simulink model "Control_Loop4_2Model"  (R2013b)
settings: Solver=ode45  StartTime=0.0  StopTime=200  RelTol=1e-3
libraries: commutil2 x756, xpclib x100, etargetslib x98, dspnetwork x98, powerlib_meascontrol x24, commcrc2 x14, dspadpt3 x4, simulink_extras x4, dspmtrx3 x4, simulink x1
(part 5 of 7)

== system Control_Loop4_2Model/GISOO-Simulation Environment/SkyMote11/Triggered Subsystem ==
  In2 : Inport
  Trigger : TriggerPort
  Byte Reversal1 : etargetslib/Byte Reversal  numInp=1
  Data Type Conversion1 : DataTypeConversion  OutDataTypeStr=uint32
  Pack : xpclib/UDP/Pack  datatypes={'uint32'}  byteAlign=1
  UDP Send : dspnetwork/UDP Send  remoteURL='127.0.0.1'  remotePort=18000+moteID  localURL='0.0.0.0'  localPortSource=Automatically determine  localPort=-1  sampletime=-1  separateLengthPort=0
  wires:
  Data Type Conversion1/1 -> Byte Reversal1/1
  Byte Reversal1/1 -> Pack/1
  Pack/1 -> UDP Send/1
  In2/1 -> Data Type Conversion1/1

== system Control_Loop4_2Model/GISOO-Simulation Environment/SkyMote11/Triggered Subsystem1 ==
  In2 : Inport
  Trigger : TriggerPort
  Byte Reversal1 : etargetslib/Byte Reversal  numInp=1
  Data Type Conversion1 : DataTypeConversion  OutDataTypeStr=uint32
  Pack : xpclib/UDP/Pack  datatypes={'uint32'}  byteAlign=1
  UDP Send : dspnetwork/UDP Send  remoteURL='127.0.0.1'  remotePort=18000+moteID  localURL='0.0.0.0'  localPortSource=Automatically determine  localPort=-1  sampletime=-1  separateLengthPort=0
  wires:
  Byte Reversal1/1 -> Pack/1
  Data Type Conversion1/1 -> Byte Reversal1/1
  In2/1 -> Data Type Conversion1/1
  Pack/1 -> UDP Send/1

== system Control_Loop4_2Model/GISOO-Simulation Environment/SkyMote11/Triggered Subsystem2 ==
  In2 : Inport
  Trigger : TriggerPort
  Byte Reversal : etargetslib/Byte Reversal  numInp=1
  Data Type Conversion1 : DataTypeConversion  OutDataTypeStr=uint32
  Pack : xpclib/UDP/Pack  datatypes={'uint32'}  byteAlign=1
  UDP Send : dspnetwork/UDP Send  remoteURL='127.0.0.1'  remotePort=18000+moteID  localURL='0.0.0.0'  localPortSource=Automatically determine  localPort=-1  sampletime=-1  separateLengthPort=0
  Out1 : Outport
  wires:
  Byte Reversal/1 -> Pack/1
  Pack/1 -> UDP Send/1
  Data Type Conversion1/1 -> Byte Reversal/1, Out1/1
  In2/1 -> Data Type Conversion1/1

== system Control_Loop4_2Model/GISOO-Simulation Environment/SkyMote11/Triggered Subsystem3 ==
  In2 : Inport
  Trigger : TriggerPort
  Byte Reversal : etargetslib/Byte Reversal  numInp=1
  Data Type Conversion1 : DataTypeConversion  OutDataTypeStr=uint32
  Pack : xpclib/UDP/Pack  datatypes={'uint32'}  byteAlign=1
  UDP Send : dspnetwork/UDP Send  remoteURL='127.0.0.1'  remotePort=18000+moteID  localURL='0.0.0.0'  localPortSource=Automatically determine  localPort=-1  sampletime=-1  separateLengthPort=0
  Out1 : Outport
  wires:
  Byte Reversal/1 -> Pack/1
  In2/1 -> Data Type Conversion1/1
  Data Type Conversion1/1 -> Out1/1, Byte Reversal/1
  Pack/1 -> UDP Send/1

== system Control_Loop4_2Model/GISOO-Simulation Environment/SkyMote11/Triggered Subsystem4 ==
  RecivedSD : Inport
  Trigger : TriggerPort
  Byte Reversal : etargetslib/Byte Reversal  numInp=1
  Constant : Constant  Value=1111
  Data Type Conversion1 : DataTypeConversion  OutDataTypeStr=uint32
  Pack : xpclib/UDP/Pack  datatypes={'uint32'}  byteAlign=1
  UDP Send : dspnetwork/UDP Send  remoteURL='127.0.0.1'  remotePort=18000+moteID  localURL='0.0.0.0'  localPortSource=Automatically determine  localPort=-1  sampletime=-1  separateLengthPort=0
  SDToApplay : Outport
  wires:
  Data Type Conversion1/1 -> Byte Reversal/1
  Byte Reversal/1 -> Pack/1
  Constant/1 -> Data Type Conversion1/1
  RecivedSD/1 -> SDToApplay/1
  Pack/1 -> UDP Send/1

== system Control_Loop4_2Model/GISOO-Simulation Environment/SkyMote11/Triggered Subsystem5 ==
  SerialDataToSend : Inport
  Trigger : TriggerPort
  Byte Reversal : etargetslib/Byte Reversal  numInp=1
  Demux : Demux  Outputs=30
  Pack : xpclib/UDP/Pack  datatypes={'uint8','uint8','uint8','uint8','uint8','uint8','uint8','uint8','uint8','uint8','uint8','uint8','uint8','uint8','uint8','uint8','uint8','uint8','uint8','uint8','uint8','uint8','uint8','uint8','uint8','uint8','uint8','uint8','uint8','uint8'}  byteAlign=1
  UDP Send : dspnetwork/UDP Send  remoteURL='127.0.0.1'  remotePort=18000+moteID  localURL='0.0.0.0'  localPortSource=Automatically determine  localPort=-1  sampletime=-1  separateLengthPort=0
  wires:
  Pack/1 -> UDP Send/1
  Demux/1 -> Pack/1
  Demux/2 -> Pack/2
  Demux/3 -> Pack/3
  Demux/4 -> Pack/4
  Demux/5 -> Pack/5
  Demux/6 -> Pack/6
  Demux/7 -> Pack/7
  Demux/8 -> Pack/8
  Demux/9 -> Pack/9
  Demux/10 -> Pack/10
  Demux/11 -> Pack/11
  Demux/12 -> Pack/12
  Demux/13 -> Pack/13
  Demux/14 -> Pack/14
  Demux/15 -> Pack/15
  Demux/16 -> Pack/16
  Demux/17 -> Pack/17
  Demux/18 -> Pack/18
  Demux/19 -> Pack/19
  Demux/20 -> Pack/20
  Demux/21 -> Pack/21
  Demux/22 -> Pack/22
  Demux/23 -> Pack/23
  Demux/24 -> Pack/24
  Demux/25 -> Pack/25
  Demux/26 -> Pack/26
  Demux/27 -> Pack/27
  Demux/28 -> Pack/28
  Demux/29 -> Pack/29
  Demux/30 -> Pack/30
  SerialDataToSend/1 -> Byte Reversal/1
  Byte Reversal/1 -> Demux/1

== system Control_Loop4_2Model/GISOO-Simulation Environment/SkyMote12/ADC0 Sender ==
  In2 : Inport
  Trigger : TriggerPort
  Byte Reversal1 : etargetslib/Byte Reversal  numInp=1
  Data Type Conversion1 : DataTypeConversion  OutDataTypeStr=uint32
  Pack : xpclib/UDP/Pack  datatypes={'uint32'}  byteAlign=1
  UDP Send : dspnetwork/UDP Send  remoteURL='127.0.0.1'  remotePort=18000+moteID  localURL='0.0.0.0'  localPortSource=Automatically determine  localPort=-1  sampletime=-1  separateLengthPort=0
  wires:
  Data Type Conversion1/1 -> Byte Reversal1/1
  Byte Reversal1/1 -> Pack/1
  In2/1 -> Data Type Conversion1/1
  Pack/1 -> UDP Send/1

== system Control_Loop4_2Model/GISOO-Simulation Environment/SkyMote12/Subsystem ==
  SerialData : Inport
  AM Packet type : Constant  Value=PacketType  OutDataTypeStr=double
  Bit to Integer Converter{,1..27} (28 alike) : commutil2/Bit to Integer Converter  nbits=8  bitOrder=MSB first  signedOutputValues=Unsigned  outDtype=Inherit via internal rule  outDtypeSigned=Inherit via internal rule
  Constant25 : Constant  Value=72  OutDataTypeStr=double
  Constant26 : Constant  Value=0  OutDataTypeStr=double
  Constant{27..30} (4 alike) : Constant  Value=255  OutDataTypeStr=double
  Constant31 : Constant  Value=16  OutDataTypeStr=double
  Constant32 : Constant  Value=137  OutDataTypeStr=double
  Demux1 : Demux  Outputs=28
  Demux2 : Demux  Outputs=16
  FrameByteEnd : Constant  Value=126  OutDataTypeStr=uint8
  FrameByteStart : Constant  Value=126  OutDataTypeStr=uint8
  Framing byte : Constant  Value=68  OutDataTypeStr=uint8
  General CRC Generator1 : commcrc2/General CRC Generator  genPoly=[1 0 0 0 1 0 0 0 0 0 0 1 0 0 0 0 1]  iniStates=0  directMethod=off  reflectInputBytes=off  reflectChecksums=off  finalXOR=0  numChecksums=1
  Integer to Bit Converter{,1..25} (26 alike) : commutil2/Integer to Bit Converter  nbits=8  signedInputValues=Unsigned  bitOrder=MSB first  outDtype=boolean
  Mux1 : Mux  Inputs=26
  Mux2 : Mux  Inputs=30
  SerialFrame : Outport
  wires:
  Bit to Integer Converter27/1 -> Mux2/3
  Demux1/28 -> Bit to Integer Converter27/1
  FrameByteStart/1 -> Mux2/30
  Bit to Integer Converter26/1 -> Mux2/2
  Demux1/27 -> Bit to Integer Converter26/1
  Demux1/15 -> Bit to Integer Converter18/1
  Demux1/14 -> Bit to Integer Converter13/1
  Demux1/6 -> Bit to Integer Converter5/1
  Demux1/16 -> Bit to Integer Converter19/1
  Demux1/25 -> Bit to Integer Converter22/1
  Demux1/17 -> Bit to Integer Converter14/1
  Demux1/18 -> Bit to Integer Converter15/1
  Demux1/26 -> Bit to Integer Converter23/1
  Demux1/22 -> Bit to Integer Converter25/1
  Demux1/23 -> Bit to Integer Converter20/1
  Demux1/20 -> Bit to Integer Converter17/1
  Demux1/19 -> Bit to Integer Converter16/1
  Demux1/5 -> Bit to Integer Converter4/1
  Demux1/21 -> Bit to Integer Converter24/1
  Demux1/4 -> Bit to Integer Converter3/1
  Demux1/24 -> Bit to Integer Converter21/1
  Constant31/1 -> Integer to Bit Converter7/1
  Integer to Bit Converter19/1 -> Mux1/20
  Integer to Bit Converter20/1 -> Mux1/21
  Integer to Bit Converter9/1 -> Mux1/10
  Integer to Bit Converter18/1 -> Mux1/19
  Demux1/12 -> Bit to Integer Converter11/1
  Mux2/1 -> SerialFrame/1
  Integer to Bit Converter12/1 -> Mux1/13
  Demux2/9 -> Integer to Bit Converter18/1
  Demux1/7 -> Bit to Integer Converter6/1
  Demux1/13 -> Bit to Integer Converter12/1
  Demux1/9 -> Bit to Integer Converter8/1
  Demux1/1 -> Bit to Integer Converter/1
  Demux2/11 -> Integer to Bit Converter20/1
  Demux1/11 -> Bit to Integer Converter10/1
  AM Packet type/1 -> Integer to Bit Converter9/1
  FrameByteEnd/1 -> Mux2/1
  Integer to Bit Converter22/1 -> Mux1/23
  Integer to Bit Converter21/1 -> Mux1/22
  Integer to Bit Converter25/1 -> Mux1/26
  Constant32/1 -> Integer to Bit Converter8/1
  Integer to Bit Converter8/1 -> Mux1/9
  General CRC Generator1/1 -> Demux1/1
  Integer to Bit Converter7/1 -> Mux1/8
  Demux1/3 -> Bit to Integer Converter2/1
  Integer to Bit Converter2/1 -> Mux1/3
  Integer to Bit Converter3/1 -> Mux1/4
  Constant28/1 -> Integer to Bit Converter4/1
  Integer to Bit Converter4/1 -> Mux1/5
  Constant27/1 -> Integer to Bit Converter3/1
  Constant26/1 -> Integer to Bit Converter2/1
  Constant29/1 -> Integer to Bit Converter5/1
  Integer to Bit Converter1/1 -> Mux1/2
  Integer to Bit Converter5/1 -> Mux1/6
  Demux2/14 -> Integer to Bit Converter23/1
  Demux2/16 -> Integer to Bit Converter25/1
  Mux1/1 -> General CRC Generator1/1
  Framing byte/1 -> Integer to Bit Converter/1
  Demux2/15 -> Integer to Bit Converter24/1
  Demux2/13 -> Integer to Bit Converter22/1
  Integer to Bit Converter/1 -> Mux1/1
  Demux2/12 -> Integer to Bit Converter21/1
  Constant25/1 -> Integer to Bit Converter1/1
  Demux2/8 -> Integer to Bit Converter17/1
  Integer to Bit Converter10/1 -> Mux1/11
  Demux2/10 -> Integer to Bit Converter19/1
  Integer to Bit Converter6/1 -> Mux1/7
  Demux1/2 -> Bit to Integer Converter1/1
  Integer to Bit Converter16/1 -> Mux1/17
  Integer to Bit Converter15/1 -> Mux1/16
  Integer to Bit Converter17/1 -> Mux1/18
  Integer to Bit Converter13/1 -> Mux1/14
  Demux1/8 -> Bit to Integer Converter7/1
  Demux1/10 -> Bit to Integer Converter9/1
  Constant30/1 -> Integer to Bit Converter6/1
  Integer to Bit Converter11/1 -> Mux1/12
  Integer to Bit Converter23/1 -> Mux1/24
  Integer to Bit Converter24/1 -> Mux1/25
  Integer to Bit Converter14/1 -> Mux1/15
  Demux2/6 -> Integer to Bit Converter15/1
  Demux2/5 -> Integer to Bit Converter14/1
  Bit to Integer Converter22/1 -> Mux2/5
  SerialData/1 -> Demux2/1
  Bit to Integer Converter21/1 -> Mux2/6
  Demux2/2 -> Integer to Bit Converter11/1
  Demux2/1 -> Integer to Bit Converter10/1
  Bit to Integer Converter17/1 -> Mux2/10
  Bit to Integer Converter20/1 -> Mux2/7
  Bit to Integer Converter/1 -> Mux2/29
  Bit to Integer Converter9/1 -> Mux2/20
  Bit to Integer Converter7/1 -> Mux2/22
  Bit to Integer Converter11/1 -> Mux2/18
  Bit to Integer Converter4/1 -> Mux2/25
  Bit to Integer Converter1/1 -> Mux2/28
  Bit to Integer Converter6/1 -> Mux2/23
  Bit to Integer Converter10/1 -> Mux2/19
  Bit to Integer Converter25/1 -> Mux2/8
  Bit to Integer Converter15/1 -> Mux2/12
  Bit to Integer Converter13/1 -> Mux2/16
  Bit to Integer Converter16/1 -> Mux2/11
  Bit to Integer Converter2/1 -> Mux2/27
  Bit to Integer Converter5/1 -> Mux2/24
  Demux2/7 -> Integer to Bit Converter16/1
  Bit to Integer Converter14/1 -> Mux2/13
  Bit to Integer Converter19/1 -> Mux2/14
  Bit to Integer Converter12/1 -> Mux2/17
  Bit to Integer Converter18/1 -> Mux2/15
  Demux2/3 -> Integer to Bit Converter12/1
  Bit to Integer Converter8/1 -> Mux2/21
  Bit to Integer Converter24/1 -> Mux2/9
  Demux2/4 -> Integer to Bit Converter13/1
  Bit to Integer Converter3/1 -> Mux2/26
  Bit to Integer Converter23/1 -> Mux2/4

== system Control_Loop4_2Model/GISOO-Simulation Environment/SkyMote12/Triggered Subsystem ==
  In2 : Inport
  Trigger : TriggerPort
  Byte Reversal1 : etargetslib/Byte Reversal  numInp=1
  Data Type Conversion1 : DataTypeConversion  OutDataTypeStr=uint32
  Pack : xpclib/UDP/Pack  datatypes={'uint32'}  byteAlign=1
  UDP Send : dspnetwork/UDP Send  remoteURL='127.0.0.1'  remotePort=18000+moteID  localURL='0.0.0.0'  localPortSource=Automatically determine  localPort=-1  sampletime=-1  separateLengthPort=0
  wires:
  Data Type Conversion1/1 -> Byte Reversal1/1
  Byte Reversal1/1 -> Pack/1
  Pack/1 -> UDP Send/1
  In2/1 -> Data Type Conversion1/1

== system Control_Loop4_2Model/GISOO-Simulation Environment/SkyMote12/Triggered Subsystem1 ==
  In2 : Inport
  Trigger : TriggerPort
  Byte Reversal1 : etargetslib/Byte Reversal  numInp=1
  Data Type Conversion1 : DataTypeConversion  OutDataTypeStr=uint32
  Pack : xpclib/UDP/Pack  datatypes={'uint32'}  byteAlign=1
  UDP Send : dspnetwork/UDP Send  remoteURL='127.0.0.1'  remotePort=18000+moteID  localURL='0.0.0.0'  localPortSource=Automatically determine  localPort=-1  sampletime=-1  separateLengthPort=0
  wires:
  Byte Reversal1/1 -> Pack/1
  Data Type Conversion1/1 -> Byte Reversal1/1
  In2/1 -> Data Type Conversion1/1
  Pack/1 -> UDP Send/1

== system Control_Loop4_2Model/GISOO-Simulation Environment/SkyMote12/Triggered Subsystem2 ==
  In2 : Inport
  Trigger : TriggerPort
  Byte Reversal : etargetslib/Byte Reversal  numInp=1
  Data Type Conversion1 : DataTypeConversion  OutDataTypeStr=uint32
  Pack : xpclib/UDP/Pack  datatypes={'uint32'}  byteAlign=1
  UDP Send : dspnetwork/UDP Send  remoteURL='127.0.0.1'  remotePort=18000+moteID  localURL='0.0.0.0'  localPortSource=Automatically determine  localPort=-1  sampletime=-1  separateLengthPort=0
  Out1 : Outport
  wires:
  Byte Reversal/1 -> Pack/1
  Pack/1 -> UDP Send/1
  Data Type Conversion1/1 -> Byte Reversal/1, Out1/1
  In2/1 -> Data Type Conversion1/1

== system Control_Loop4_2Model/GISOO-Simulation Environment/SkyMote12/Triggered Subsystem3 ==
  In2 : Inport
  Trigger : TriggerPort
  Byte Reversal : etargetslib/Byte Reversal  numInp=1
  Data Type Conversion1 : DataTypeConversion  OutDataTypeStr=uint32
  Pack : xpclib/UDP/Pack  datatypes={'uint32'}  byteAlign=1
  UDP Send : dspnetwork/UDP Send  remoteURL='127.0.0.1'  remotePort=18000+moteID  localURL='0.0.0.0'  localPortSource=Automatically determine  localPort=-1  sampletime=-1  separateLengthPort=0
  Out1 : Outport
  wires:
  Byte Reversal/1 -> Pack/1
  In2/1 -> Data Type Conversion1/1
  Data Type Conversion1/1 -> Out1/1, Byte Reversal/1
  Pack/1 -> UDP Send/1

== system Control_Loop4_2Model/GISOO-Simulation Environment/SkyMote12/Triggered Subsystem4 ==
  RecivedSD : Inport
  Trigger : TriggerPort
  Byte Reversal : etargetslib/Byte Reversal  numInp=1
  Constant : Constant  Value=1111
  Data Type Conversion1 : DataTypeConversion  OutDataTypeStr=uint32
  Pack : xpclib/UDP/Pack  datatypes={'uint32'}  byteAlign=1
  UDP Send : dspnetwork/UDP Send  remoteURL='127.0.0.1'  remotePort=18000+moteID  localURL='0.0.0.0'  localPortSource=Automatically determine  localPort=-1  sampletime=-1  separateLengthPort=0
  SDToApplay : Outport
  wires:
  Data Type Conversion1/1 -> Byte Reversal/1
  Byte Reversal/1 -> Pack/1
  Constant/1 -> Data Type Conversion1/1
  RecivedSD/1 -> SDToApplay/1
  Pack/1 -> UDP Send/1

== system Control_Loop4_2Model/GISOO-Simulation Environment/SkyMote12/Triggered Subsystem5 ==
  SerialDataToSend : Inport
  Trigger : TriggerPort
  Byte Reversal : etargetslib/Byte Reversal  numInp=1
  Demux : Demux  Outputs=30
  Pack : xpclib/UDP/Pack  datatypes={'uint8','uint8','uint8','uint8','uint8','uint8','uint8','uint8','uint8','uint8','uint8','uint8','uint8','uint8','uint8','uint8','uint8','uint8','uint8','uint8','uint8','uint8','uint8','uint8','uint8','uint8','uint8','uint8','uint8','uint8'}  byteAlign=1
  UDP Send : dspnetwork/UDP Send  remoteURL='127.0.0.1'  remotePort=18000+moteID  localURL='0.0.0.0'  localPortSource=Automatically determine  localPort=-1  sampletime=-1  separateLengthPort=0
  wires:
  Pack/1 -> UDP Send/1
  Demux/1 -> Pack/1
  Demux/2 -> Pack/2
  Demux/3 -> Pack/3
  Demux/4 -> Pack/4
  Demux/5 -> Pack/5
  Demux/6 -> Pack/6
  Demux/7 -> Pack/7
  Demux/8 -> Pack/8
  Demux/9 -> Pack/9
  Demux/10 -> Pack/10
  Demux/11 -> Pack/11
  Demux/12 -> Pack/12
  Demux/13 -> Pack/13
  Demux/14 -> Pack/14
  Demux/15 -> Pack/15
  Demux/16 -> Pack/16
  Demux/17 -> Pack/17
  Demux/18 -> Pack/18
  Demux/19 -> Pack/19
  Demux/20 -> Pack/20
  Demux/21 -> Pack/21
  Demux/22 -> Pack/22
  Demux/23 -> Pack/23
  Demux/24 -> Pack/24
  Demux/25 -> Pack/25
  Demux/26 -> Pack/26
  Demux/27 -> Pack/27
  Demux/28 -> Pack/28
  Demux/29 -> Pack/29
  Demux/30 -> Pack/30
  SerialDataToSend/1 -> Byte Reversal/1
  Byte Reversal/1 -> Demux/1

== system Control_Loop4_2Model/GISOO-Simulation Environment/SkyMote13/ADC0 Sender ==
  In2 : Inport
  Trigger : TriggerPort
  Byte Reversal1 : etargetslib/Byte Reversal  numInp=1
  Data Type Conversion1 : DataTypeConversion  OutDataTypeStr=uint32
  Pack : xpclib/UDP/Pack  datatypes={'uint32'}  byteAlign=1
  UDP Send : dspnetwork/UDP Send  remoteURL='127.0.0.1'  remotePort=18000+moteID  localURL='0.0.0.0'  localPortSource=Automatically determine  localPort=-1  sampletime=-1  separateLengthPort=0
  wires:
  Data Type Conversion1/1 -> Byte Reversal1/1
  Byte Reversal1/1 -> Pack/1
  In2/1 -> Data Type Conversion1/1
  Pack/1 -> UDP Send/1

== system Control_Loop4_2Model/GISOO-Simulation Environment/SkyMote13/Subsystem ==
  SerialData : Inport
  AM Packet type : Constant  Value=PacketType  OutDataTypeStr=double
  Bit to Integer Converter{,1..27} (28 alike) : commutil2/Bit to Integer Converter  nbits=8  bitOrder=MSB first  signedOutputValues=Unsigned  outDtype=Inherit via internal rule  outDtypeSigned=Inherit via internal rule
  Constant25 : Constant  Value=72  OutDataTypeStr=double
  Constant26 : Constant  Value=0  OutDataTypeStr=double
  Constant{27..30} (4 alike) : Constant  Value=255  OutDataTypeStr=double
  Constant31 : Constant  Value=16  OutDataTypeStr=double
  Constant32 : Constant  Value=137  OutDataTypeStr=double
  Demux1 : Demux  Outputs=28
  Demux2 : Demux  Outputs=16
  FrameByteEnd : Constant  Value=126  OutDataTypeStr=uint8
  FrameByteStart : Constant  Value=126  OutDataTypeStr=uint8
  Framing byte : Constant  Value=68  OutDataTypeStr=uint8
  General CRC Generator1 : commcrc2/General CRC Generator  genPoly=[1 0 0 0 1 0 0 0 0 0 0 1 0 0 0 0 1]  iniStates=0  directMethod=off  reflectInputBytes=off  reflectChecksums=off  finalXOR=0  numChecksums=1
  Integer to Bit Converter{,1..25} (26 alike) : commutil2/Integer to Bit Converter  nbits=8  signedInputValues=Unsigned  bitOrder=MSB first  outDtype=boolean
  Mux1 : Mux  Inputs=26
  Mux2 : Mux  Inputs=30
  SerialFrame : Outport
  wires:
  Bit to Integer Converter27/1 -> Mux2/3
  Demux1/28 -> Bit to Integer Converter27/1
  FrameByteStart/1 -> Mux2/30
  Bit to Integer Converter26/1 -> Mux2/2
  Demux1/27 -> Bit to Integer Converter26/1
  Demux1/15 -> Bit to Integer Converter18/1
  Demux1/14 -> Bit to Integer Converter13/1
  Demux1/6 -> Bit to Integer Converter5/1
  Demux1/16 -> Bit to Integer Converter19/1
  Demux1/25 -> Bit to Integer Converter22/1
  Demux1/17 -> Bit to Integer Converter14/1
  Demux1/18 -> Bit to Integer Converter15/1
  Demux1/26 -> Bit to Integer Converter23/1
  Demux1/22 -> Bit to Integer Converter25/1
  Demux1/23 -> Bit to Integer Converter20/1
  Demux1/20 -> Bit to Integer Converter17/1
  Demux1/19 -> Bit to Integer Converter16/1
  Demux1/5 -> Bit to Integer Converter4/1
  Demux1/21 -> Bit to Integer Converter24/1
  Demux1/4 -> Bit to Integer Converter3/1
  Demux1/24 -> Bit to Integer Converter21/1
  Constant31/1 -> Integer to Bit Converter7/1
  Integer to Bit Converter19/1 -> Mux1/20
  Integer to Bit Converter20/1 -> Mux1/21
  Integer to Bit Converter9/1 -> Mux1/10
  Integer to Bit Converter18/1 -> Mux1/19
  Demux1/12 -> Bit to Integer Converter11/1
  Mux2/1 -> SerialFrame/1
  Integer to Bit Converter12/1 -> Mux1/13
  Demux2/9 -> Integer to Bit Converter18/1
  Demux1/7 -> Bit to Integer Converter6/1
  Demux1/13 -> Bit to Integer Converter12/1
  Demux1/9 -> Bit to Integer Converter8/1
  Demux1/1 -> Bit to Integer Converter/1
  Demux2/11 -> Integer to Bit Converter20/1
  Demux1/11 -> Bit to Integer Converter10/1
  AM Packet type/1 -> Integer to Bit Converter9/1
  FrameByteEnd/1 -> Mux2/1
  Integer to Bit Converter22/1 -> Mux1/23
  Integer to Bit Converter21/1 -> Mux1/22
  Integer to Bit Converter25/1 -> Mux1/26
  Constant32/1 -> Integer to Bit Converter8/1
  Integer to Bit Converter8/1 -> Mux1/9
  General CRC Generator1/1 -> Demux1/1
  Integer to Bit Converter7/1 -> Mux1/8
  Demux1/3 -> Bit to Integer Converter2/1
  Integer to Bit Converter2/1 -> Mux1/3
  Integer to Bit Converter3/1 -> Mux1/4
  Constant28/1 -> Integer to Bit Converter4/1
  Integer to Bit Converter4/1 -> Mux1/5
  Constant27/1 -> Integer to Bit Converter3/1
  Constant26/1 -> Integer to Bit Converter2/1
  Constant29/1 -> Integer to Bit Converter5/1
  Integer to Bit Converter1/1 -> Mux1/2
  Integer to Bit Converter5/1 -> Mux1/6
  Demux2/14 -> Integer to Bit Converter23/1
  Demux2/16 -> Integer to Bit Converter25/1
  Mux1/1 -> General CRC Generator1/1
  Framing byte/1 -> Integer to Bit Converter/1
  Demux2/15 -> Integer to Bit Converter24/1
  Demux2/13 -> Integer to Bit Converter22/1
  Integer to Bit Converter/1 -> Mux1/1
  Demux2/12 -> Integer to Bit Converter21/1
  Constant25/1 -> Integer to Bit Converter1/1
  Demux2/8 -> Integer to Bit Converter17/1
  Integer to Bit Converter10/1 -> Mux1/11
  Demux2/10 -> Integer to Bit Converter19/1
  Integer to Bit Converter6/1 -> Mux1/7
  Demux1/2 -> Bit to Integer Converter1/1
  Integer to Bit Converter16/1 -> Mux1/17
  Integer to Bit Converter15/1 -> Mux1/16
  Integer to Bit Converter17/1 -> Mux1/18
  Integer to Bit Converter13/1 -> Mux1/14
  Demux1/8 -> Bit to Integer Converter7/1
  Demux1/10 -> Bit to Integer Converter9/1
  Constant30/1 -> Integer to Bit Converter6/1
  Integer to Bit Converter11/1 -> Mux1/12
  Integer to Bit Converter23/1 -> Mux1/24
  Integer to Bit Converter24/1 -> Mux1/25
  Integer to Bit Converter14/1 -> Mux1/15
  Demux2/6 -> Integer to Bit Converter15/1
  Demux2/5 -> Integer to Bit Converter14/1
  Bit to Integer Converter22/1 -> Mux2/5
  SerialData/1 -> Demux2/1
  Bit to Integer Converter21/1 -> Mux2/6
  Demux2/2 -> Integer to Bit Converter11/1
  Demux2/1 -> Integer to Bit Converter10/1
  Bit to Integer Converter17/1 -> Mux2/10
  Bit to Integer Converter20/1 -> Mux2/7
  Bit to Integer Converter/1 -> Mux2/29
  Bit to Integer Converter9/1 -> Mux2/20
  Bit to Integer Converter7/1 -> Mux2/22
  Bit to Integer Converter11/1 -> Mux2/18
  Bit to Integer Converter4/1 -> Mux2/25
  Bit to Integer Converter1/1 -> Mux2/28
  Bit to Integer Converter6/1 -> Mux2/23
  Bit to Integer Converter10/1 -> Mux2/19
  Bit to Integer Converter25/1 -> Mux2/8
  Bit to Integer Converter15/1 -> Mux2/12
  Bit to Integer Converter13/1 -> Mux2/16
  Bit to Integer Converter16/1 -> Mux2/11
  Bit to Integer Converter2/1 -> Mux2/27
  Bit to Integer Converter5/1 -> Mux2/24
  Demux2/7 -> Integer to Bit Converter16/1
  Bit to Integer Converter14/1 -> Mux2/13
  Bit to Integer Converter19/1 -> Mux2/14
  Bit to Integer Converter12/1 -> Mux2/17
  Bit to Integer Converter18/1 -> Mux2/15
  Demux2/3 -> Integer to Bit Converter12/1
  Bit to Integer Converter8/1 -> Mux2/21
  Bit to Integer Converter24/1 -> Mux2/9
  Demux2/4 -> Integer to Bit Converter13/1
  Bit to Integer Converter3/1 -> Mux2/26
  Bit to Integer Converter23/1 -> Mux2/4

== system Control_Loop4_2Model/GISOO-Simulation Environment/SkyMote13/Triggered Subsystem ==
  In2 : Inport
  Trigger : TriggerPort
  Byte Reversal1 : etargetslib/Byte Reversal  numInp=1
  Data Type Conversion1 : DataTypeConversion  OutDataTypeStr=uint32
  Pack : xpclib/UDP/Pack  datatypes={'uint32'}  byteAlign=1
  UDP Send : dspnetwork/UDP Send  remoteURL='127.0.0.1'  remotePort=18000+moteID  localURL='0.0.0.0'  localPortSource=Automatically determine  localPort=-1  sampletime=-1  separateLengthPort=0
  wires:
  Data Type Conversion1/1 -> Byte Reversal1/1
  Byte Reversal1/1 -> Pack/1
  Pack/1 -> UDP Send/1
  In2/1 -> Data Type Conversion1/1

== system Control_Loop4_2Model/GISOO-Simulation Environment/SkyMote13/Triggered Subsystem1 ==
  In2 : Inport
  Trigger : TriggerPort
  Byte Reversal1 : etargetslib/Byte Reversal  numInp=1
  Data Type Conversion1 : DataTypeConversion  OutDataTypeStr=uint32
  Pack : xpclib/UDP/Pack  datatypes={'uint32'}  byteAlign=1
  UDP Send : dspnetwork/UDP Send  remoteURL='127.0.0.1'  remotePort=18000+moteID  localURL='0.0.0.0'  localPortSource=Automatically determine  localPort=-1  sampletime=-1  separateLengthPort=0
  wires:
  Byte Reversal1/1 -> Pack/1
  Data Type Conversion1/1 -> Byte Reversal1/1
  In2/1 -> Data Type Conversion1/1
  Pack/1 -> UDP Send/1

== system Control_Loop4_2Model/GISOO-Simulation Environment/SkyMote13/Triggered Subsystem2 ==
  In2 : Inport
  Trigger : TriggerPort
  Byte Reversal : etargetslib/Byte Reversal  numInp=1
  Data Type Conversion1 : DataTypeConversion  OutDataTypeStr=uint32
  Pack : xpclib/UDP/Pack  datatypes={'uint32'}  byteAlign=1
  UDP Send : dspnetwork/UDP Send  remoteURL='127.0.0.1'  remotePort=18000+moteID  localURL='0.0.0.0'  localPortSource=Automatically determine  localPort=-1  sampletime=-1  separateLengthPort=0
  Out1 : Outport
  wires:
  Byte Reversal/1 -> Pack/1
  Pack/1 -> UDP Send/1
  Data Type Conversion1/1 -> Byte Reversal/1, Out1/1
  In2/1 -> Data Type Conversion1/1

== system Control_Loop4_2Model/GISOO-Simulation Environment/SkyMote13/Triggered Subsystem3 ==
  In2 : Inport
  Trigger : TriggerPort
  Byte Reversal : etargetslib/Byte Reversal  numInp=1
  Data Type Conversion1 : DataTypeConversion  OutDataTypeStr=uint32
  Pack : xpclib/UDP/Pack  datatypes={'uint32'}  byteAlign=1
  UDP Send : dspnetwork/UDP Send  remoteURL='127.0.0.1'  remotePort=18000+moteID  localURL='0.0.0.0'  localPortSource=Automatically determine  localPort=-1  sampletime=-1  separateLengthPort=0
  Out1 : Outport
  wires:
  Byte Reversal/1 -> Pack/1
  In2/1 -> Data Type Conversion1/1
  Data Type Conversion1/1 -> Out1/1, Byte Reversal/1
  Pack/1 -> UDP Send/1

== system Control_Loop4_2Model/GISOO-Simulation Environment/SkyMote13/Triggered Subsystem4 ==
  RecivedSD : Inport
  Trigger : TriggerPort
  Byte Reversal : etargetslib/Byte Reversal  numInp=1
  Constant : Constant  Value=1111
  Data Type Conversion1 : DataTypeConversion  OutDataTypeStr=uint32
  Pack : xpclib/UDP/Pack  datatypes={'uint32'}  byteAlign=1
  UDP Send : dspnetwork/UDP Send  remoteURL='127.0.0.1'  remotePort=18000+moteID  localURL='0.0.0.0'  localPortSource=Automatically determine  localPort=-1  sampletime=-1  separateLengthPort=0
  SDToApplay : Outport
  wires:
  Data Type Conversion1/1 -> Byte Reversal/1
  Byte Reversal/1 -> Pack/1
  Constant/1 -> Data Type Conversion1/1
  RecivedSD/1 -> SDToApplay/1
  Pack/1 -> UDP Send/1

== system Control_Loop4_2Model/GISOO-Simulation Environment/SkyMote13/Triggered Subsystem5 ==
  SerialDataToSend : Inport
  Trigger : TriggerPort
  Byte Reversal : etargetslib/Byte Reversal  numInp=1
  Demux : Demux  Outputs=30
  Pack : xpclib/UDP/Pack  datatypes={'uint8','uint8','uint8','uint8','uint8','uint8','uint8','uint8','uint8','uint8','uint8','uint8','uint8','uint8','uint8','uint8','uint8','uint8','uint8','uint8','uint8','uint8','uint8','uint8','uint8','uint8','uint8','uint8','uint8','uint8'}  byteAlign=1
  UDP Send : dspnetwork/UDP Send  remoteURL='127.0.0.1'  remotePort=18000+moteID  localURL='0.0.0.0'  localPortSource=Automatically determine  localPort=-1  sampletime=-1  separateLengthPort=0
  wires:
  Pack/1 -> UDP Send/1
  Demux/1 -> Pack/1
  Demux/2 -> Pack/2
  Demux/3 -> Pack/3
  Demux/4 -> Pack/4
  Demux/5 -> Pack/5
  Demux/6 -> Pack/6
  Demux/7 -> Pack/7
  Demux/8 -> Pack/8
  Demux/9 -> Pack/9
  Demux/10 -> Pack/10
  Demux/11 -> Pack/11
  Demux/12 -> Pack/12
  Demux/13 -> Pack/13
  Demux/14 -> Pack/14
  Demux/15 -> Pack/15
  Demux/16 -> Pack/16
  Demux/17 -> Pack/17
  Demux/18 -> Pack/18
  Demux/19 -> Pack/19
  Demux/20 -> Pack/20
  Demux/21 -> Pack/21
  Demux/22 -> Pack/22
  Demux/23 -> Pack/23
  Demux/24 -> Pack/24
  Demux/25 -> Pack/25
  Demux/26 -> Pack/26
  Demux/27 -> Pack/27
  Demux/28 -> Pack/28
  Demux/29 -> Pack/29
  Demux/30 -> Pack/30
  SerialDataToSend/1 -> Byte Reversal/1
  Byte Reversal/1 -> Demux/1

== system Control_Loop4_2Model/GISOO-Simulation Environment/SkyMote2/ADC0 Sender ==
  In2 : Inport
  Trigger : TriggerPort
  Byte Reversal1 : etargetslib/Byte Reversal  numInp=1
  Data Type Conversion1 : DataTypeConversion  OutDataTypeStr=uint32
  Pack : xpclib/UDP/Pack  datatypes={'uint32'}  byteAlign=1
  UDP Send : dspnetwork/UDP Send  remoteURL='127.0.0.1'  remotePort=18000+moteID  localURL='0.0.0.0'  localPortSource=Automatically determine  localPort=-1  sampletime=-1  separateLengthPort=0
  wires:
  Data Type Conversion1/1 -> Byte Reversal1/1
  Byte Reversal1/1 -> Pack/1
  In2/1 -> Data Type Conversion1/1
  Pack/1 -> UDP Send/1

== system Control_Loop4_2Model/GISOO-Simulation Environment/SkyMote2/Subsystem ==
  SerialData : Inport
  AM Packet type : Constant  Value=PacketType  OutDataTypeStr=double
  Bit to Integer Converter{,1..27} (28 alike) : commutil2/Bit to Integer Converter  nbits=8  bitOrder=MSB first  signedOutputValues=Unsigned  outDtype=Inherit via internal rule  outDtypeSigned=Inherit via internal rule
  Constant25 : Constant  Value=72  OutDataTypeStr=double
  Constant26 : Constant  Value=0  OutDataTypeStr=double
  Constant{27..30} (4 alike) : Constant  Value=255  OutDataTypeStr=double
  Constant31 : Constant  Value=16  OutDataTypeStr=double
  Constant32 : Constant  Value=137  OutDataTypeStr=double
  Demux1 : Demux  Outputs=28
  Demux2 : Demux  Outputs=16
  FrameByteEnd : Constant  Value=126  OutDataTypeStr=uint8
  FrameByteStart : Constant  Value=126  OutDataTypeStr=uint8
  Framing byte : Constant  Value=68  OutDataTypeStr=uint8
  General CRC Generator1 : commcrc2/General CRC Generator  genPoly=[1 0 0 0 1 0 0 0 0 0 0 1 0 0 0 0 1]  iniStates=0  directMethod=off  reflectInputBytes=off  reflectChecksums=off  finalXOR=0  numChecksums=1
  Integer to Bit Converter{,1..25} (26 alike) : commutil2/Integer to Bit Converter  nbits=8  signedInputValues=Unsigned  bitOrder=MSB first  outDtype=boolean
  Mux1 : Mux  Inputs=26
  Mux2 : Mux  Inputs=30
  SerialFrame : Outport
  wires:
  Bit to Integer Converter27/1 -> Mux2/3
  Demux1/28 -> Bit to Integer Converter27/1
  FrameByteStart/1 -> Mux2/30
  Bit to Integer Converter26/1 -> Mux2/2
  Demux1/27 -> Bit to Integer Converter26/1
  Demux1/15 -> Bit to Integer Converter18/1
  Demux1/14 -> Bit to Integer Converter13/1
  Demux1/6 -> Bit to Integer Converter5/1
  Demux1/16 -> Bit to Integer Converter19/1
  Demux1/25 -> Bit to Integer Converter22/1
  Demux1/17 -> Bit to Integer Converter14/1
  Demux1/18 -> Bit to Integer Converter15/1
  Demux1/26 -> Bit to Integer Converter23/1
  Demux1/22 -> Bit to Integer Converter25/1
  Demux1/23 -> Bit to Integer Converter20/1
  Demux1/20 -> Bit to Integer Converter17/1
  Demux1/19 -> Bit to Integer Converter16/1
  Demux1/5 -> Bit to Integer Converter4/1
  Demux1/21 -> Bit to Integer Converter24/1
  Demux1/4 -> Bit to Integer Converter3/1
  Demux1/24 -> Bit to Integer Converter21/1
  Constant31/1 -> Integer to Bit Converter7/1
  Integer to Bit Converter19/1 -> Mux1/20
  Integer to Bit Converter20/1 -> Mux1/21
  Integer to Bit Converter9/1 -> Mux1/10
  Integer to Bit Converter18/1 -> Mux1/19
  Demux1/12 -> Bit to Integer Converter11/1
  Mux2/1 -> SerialFrame/1
  Integer to Bit Converter12/1 -> Mux1/13
  Demux2/9 -> Integer to Bit Converter18/1
  Demux1/7 -> Bit to Integer Converter6/1
  Demux1/13 -> Bit to Integer Converter12/1
  Demux1/9 -> Bit to Integer Converter8/1
  Demux1/1 -> Bit to Integer Converter/1
  Demux2/11 -> Integer to Bit Converter20/1
  Demux1/11 -> Bit to Integer Converter10/1
  AM Packet type/1 -> Integer to Bit Converter9/1
  FrameByteEnd/1 -> Mux2/1
  Integer to Bit Converter22/1 -> Mux1/23
  Integer to Bit Converter21/1 -> Mux1/22
  Integer to Bit Converter25/1 -> Mux1/26
  Constant32/1 -> Integer to Bit Converter8/1
  Integer to Bit Converter8/1 -> Mux1/9
  General CRC Generator1/1 -> Demux1/1
  Integer to Bit Converter7/1 -> Mux1/8
  Demux1/3 -> Bit to Integer Converter2/1
  Integer to Bit Converter2/1 -> Mux1/3
  Integer to Bit Converter3/1 -> Mux1/4
  Constant28/1 -> Integer to Bit Converter4/1
  Integer to Bit Converter4/1 -> Mux1/5
  Constant27/1 -> Integer to Bit Converter3/1
  Constant26/1 -> Integer to Bit Converter2/1
  Constant29/1 -> Integer to Bit Converter5/1
  Integer to Bit Converter1/1 -> Mux1/2
  Integer to Bit Converter5/1 -> Mux1/6
  Demux2/14 -> Integer to Bit Converter23/1
  Demux2/16 -> Integer to Bit Converter25/1
  Mux1/1 -> General CRC Generator1/1
  Framing byte/1 -> Integer to Bit Converter/1
  Demux2/15 -> Integer to Bit Converter24/1
  Demux2/13 -> Integer to Bit Converter22/1
  Integer to Bit Converter/1 -> Mux1/1
  Demux2/12 -> Integer to Bit Converter21/1
  Constant25/1 -> Integer to Bit Converter1/1
  Demux2/8 -> Integer to Bit Converter17/1
  Integer to Bit Converter10/1 -> Mux1/11
  Demux2/10 -> Integer to Bit Converter19/1
  Integer to Bit Converter6/1 -> Mux1/7
  Demux1/2 -> Bit to Integer Converter1/1
  Integer to Bit Converter16/1 -> Mux1/17
  Integer to Bit Converter15/1 -> Mux1/16
  Integer to Bit Converter17/1 -> Mux1/18
  Integer to Bit Converter13/1 -> Mux1/14
  Demux1/8 -> Bit to Integer Converter7/1
  Demux1/10 -> Bit to Integer Converter9/1
  Constant30/1 -> Integer to Bit Converter6/1
  Integer to Bit Converter11/1 -> Mux1/12
  Integer to Bit Converter23/1 -> Mux1/24
  Integer to Bit Converter24/1 -> Mux1/25
  Integer to Bit Converter14/1 -> Mux1/15
  Demux2/6 -> Integer to Bit Converter15/1
  Demux2/5 -> Integer to Bit Converter14/1
  Bit to Integer Converter22/1 -> Mux2/5
  SerialData/1 -> Demux2/1
  Bit to Integer Converter21/1 -> Mux2/6
  Demux2/2 -> Integer to Bit Converter11/1
  Demux2/1 -> Integer to Bit Converter10/1
  Bit to Integer Converter17/1 -> Mux2/10
  Bit to Integer Converter20/1 -> Mux2/7
  Bit to Integer Converter/1 -> Mux2/29
  Bit to Integer Converter9/1 -> Mux2/20
  Bit to Integer Converter7/1 -> Mux2/22
  Bit to Integer Converter11/1 -> Mux2/18
  Bit to Integer Converter4/1 -> Mux2/25
  Bit to Integer Converter1/1 -> Mux2/28
  Bit to Integer Converter6/1 -> Mux2/23
  Bit to Integer Converter10/1 -> Mux2/19
  Bit to Integer Converter25/1 -> Mux2/8
  Bit to Integer Converter15/1 -> Mux2/12
  Bit to Integer Converter13/1 -> Mux2/16
  Bit to Integer Converter16/1 -> Mux2/11
  Bit to Integer Converter2/1 -> Mux2/27
  Bit to Integer Converter5/1 -> Mux2/24
  Demux2/7 -> Integer to Bit Converter16/1
  Bit to Integer Converter14/1 -> Mux2/13
  Bit to Integer Converter19/1 -> Mux2/14
  Bit to Integer Converter12/1 -> Mux2/17
  Bit to Integer Converter18/1 -> Mux2/15
  Demux2/3 -> Integer to Bit Converter12/1
  Bit to Integer Converter8/1 -> Mux2/21
  Bit to Integer Converter24/1 -> Mux2/9
  Demux2/4 -> Integer to Bit Converter13/1
  Bit to Integer Converter3/1 -> Mux2/26
  Bit to Integer Converter23/1 -> Mux2/4

== system Control_Loop4_2Model/GISOO-Simulation Environment/SkyMote2/Triggered Subsystem ==
  In2 : Inport
  Trigger : TriggerPort
  Byte Reversal1 : etargetslib/Byte Reversal  numInp=1
  Data Type Conversion1 : DataTypeConversion  OutDataTypeStr=uint32
  Pack : xpclib/UDP/Pack  datatypes={'uint32'}  byteAlign=1
  UDP Send : dspnetwork/UDP Send  remoteURL='127.0.0.1'  remotePort=18000+moteID  localURL='0.0.0.0'  localPortSource=Automatically determine  localPort=-1  sampletime=-1  separateLengthPort=0
  wires:
  Data Type Conversion1/1 -> Byte Reversal1/1
  Byte Reversal1/1 -> Pack/1
  Pack/1 -> UDP Send/1
  In2/1 -> Data Type Conversion1/1

== system Control_Loop4_2Model/GISOO-Simulation Environment/SkyMote2/Triggered Subsystem1 ==
  In2 : Inport
  Trigger : TriggerPort
  Byte Reversal1 : etargetslib/Byte Reversal  numInp=1
  Data Type Conversion1 : DataTypeConversion  OutDataTypeStr=uint32
  Pack : xpclib/UDP/Pack  datatypes={'uint32'}  byteAlign=1
  UDP Send : dspnetwork/UDP Send  remoteURL='127.0.0.1'  remotePort=18000+moteID  localURL='0.0.0.0'  localPortSource=Automatically determine  localPort=-1  sampletime=-1  separateLengthPort=0
  wires:
  Byte Reversal1/1 -> Pack/1
  Data Type Conversion1/1 -> Byte Reversal1/1
  In2/1 -> Data Type Conversion1/1
  Pack/1 -> UDP Send/1

== system Control_Loop4_2Model/GISOO-Simulation Environment/SkyMote2/Triggered Subsystem2 ==
  In2 : Inport
  Trigger : TriggerPort
  Byte Reversal : etargetslib/Byte Reversal  numInp=1
  Data Type Conversion1 : DataTypeConversion  OutDataTypeStr=uint32
  Pack : xpclib/UDP/Pack  datatypes={'uint32'}  byteAlign=1
  UDP Send : dspnetwork/UDP Send  remoteURL='127.0.0.1'  remotePort=18000+moteID  localURL='0.0.0.0'  localPortSource=Automatically determine  localPort=-1  sampletime=-1  separateLengthPort=0
  Out1 : Outport
  wires:
  Byte Reversal/1 -> Pack/1
  Pack/1 -> UDP Send/1
  Data Type Conversion1/1 -> Byte Reversal/1, Out1/1
  In2/1 -> Data Type Conversion1/1

== system Control_Loop4_2Model/GISOO-Simulation Environment/SkyMote2/Triggered Subsystem3 ==
  In2 : Inport
  Trigger : TriggerPort
  Byte Reversal : etargetslib/Byte Reversal  numInp=1
  Data Type Conversion1 : DataTypeConversion  OutDataTypeStr=uint32
  Pack : xpclib/UDP/Pack  datatypes={'uint32'}  byteAlign=1
  UDP Send : dspnetwork/UDP Send  remoteURL='127.0.0.1'  remotePort=18000+moteID  localURL='0.0.0.0'  localPortSource=Automatically determine  localPort=-1  sampletime=-1  separateLengthPort=0
  Out1 : Outport
  wires:
  Byte Reversal/1 -> Pack/1
  In2/1 -> Data Type Conversion1/1
  Data Type Conversion1/1 -> Out1/1, Byte Reversal/1
  Pack/1 -> UDP Send/1

== system Control_Loop4_2Model/GISOO-Simulation Environment/SkyMote2/Triggered Subsystem4 ==
  RecivedSD : Inport
  Trigger : TriggerPort
  Byte Reversal : etargetslib/Byte Reversal  numInp=1
  Constant : Constant  Value=1111
  Data Type Conversion1 : DataTypeConversion  OutDataTypeStr=uint32
  Pack : xpclib/UDP/Pack  datatypes={'uint32'}  byteAlign=1
  UDP Send : dspnetwork/UDP Send  remoteURL='127.0.0.1'  remotePort=18000+moteID  localURL='0.0.0.0'  localPortSource=Automatically determine  localPort=-1  sampletime=-1  separateLengthPort=0
  SDToApplay : Outport
  wires:
  Data Type Conversion1/1 -> Byte Reversal/1
  Byte Reversal/1 -> Pack/1
  Constant/1 -> Data Type Conversion1/1
  RecivedSD/1 -> SDToApplay/1
  Pack/1 -> UDP Send/1

== system Control_Loop4_2Model/GISOO-Simulation Environment/SkyMote2/Triggered Subsystem5 ==
  SerialDataToSend : Inport
  Trigger : TriggerPort
  Byte Reversal : etargetslib/Byte Reversal  numInp=1
  Demux : Demux  Outputs=30
  Pack : xpclib/UDP/Pack  datatypes={'uint8','uint8','uint8','uint8','uint8','uint8','uint8','uint8','uint8','uint8','uint8','uint8','uint8','uint8','uint8','uint8','uint8','uint8','uint8','uint8','uint8','uint8','uint8','uint8','uint8','uint8','uint8','uint8','uint8','uint8'}  byteAlign=1
  UDP Send : dspnetwork/UDP Send  remoteURL='127.0.0.1'  remotePort=18000+moteID  localURL='0.0.0.0'  localPortSource=Automatically determine  localPort=-1  sampletime=-1  separateLengthPort=0
  wires:
  Pack/1 -> UDP Send/1
  Demux/1 -> Pack/1
  Demux/2 -> Pack/2
  Demux/3 -> Pack/3
  Demux/4 -> Pack/4
  Demux/5 -> Pack/5
  Demux/6 -> Pack/6
  Demux/7 -> Pack/7
  Demux/8 -> Pack/8
  Demux/9 -> Pack/9
  Demux/10 -> Pack/10
  Demux/11 -> Pack/11
  Demux/12 -> Pack/12
  Demux/13 -> Pack/13
  Demux/14 -> Pack/14
  Demux/15 -> Pack/15
  Demux/16 -> Pack/16
  Demux/17 -> Pack/17
  Demux/18 -> Pack/18
  Demux/19 -> Pack/19
  Demux/20 -> Pack/20
  Demux/21 -> Pack/21
  Demux/22 -> Pack/22
  Demux/23 -> Pack/23
  Demux/24 -> Pack/24
  Demux/25 -> Pack/25
  Demux/26 -> Pack/26
  Demux/27 -> Pack/27
  Demux/28 -> Pack/28
  Demux/29 -> Pack/29
  Demux/30 -> Pack/30
  SerialDataToSend/1 -> Byte Reversal/1
  Byte Reversal/1 -> Demux/1

== system Control_Loop4_2Model/GISOO-Simulation Environment/SkyMote3/ADC0 Sender ==
  In2 : Inport
  Trigger : TriggerPort
  Byte Reversal1 : etargetslib/Byte Reversal  numInp=1
  Data Type Conversion1 : DataTypeConversion  OutDataTypeStr=uint32
  Pack : xpclib/UDP/Pack  datatypes={'uint32'}  byteAlign=1
  UDP Send : dspnetwork/UDP Send  remoteURL='127.0.0.1'  remotePort=18000+moteID  localURL='0.0.0.0'  localPortSource=Automatically determine  localPort=-1  sampletime=-1  separateLengthPort=0
  wires:
  Data Type Conversion1/1 -> Byte Reversal1/1
  Byte Reversal1/1 -> Pack/1
  In2/1 -> Data Type Conversion1/1
  Pack/1 -> UDP Send/1

== system Control_Loop4_2Model/GISOO-Simulation Environment/SkyMote3/Subsystem ==
  SerialData : Inport
  AM Packet type : Constant  Value=PacketType  OutDataTypeStr=double
  Bit to Integer Converter{,1..27} (28 alike) : commutil2/Bit to Integer Converter  nbits=8  bitOrder=MSB first  signedOutputValues=Unsigned  outDtype=Inherit via internal rule  outDtypeSigned=Inherit via internal rule
  Constant25 : Constant  Value=72  OutDataTypeStr=double
  Constant26 : Constant  Value=0  OutDataTypeStr=double
  Constant{27..30} (4 alike) : Constant  Value=255  OutDataTypeStr=double
  Constant31 : Constant  Value=16  OutDataTypeStr=double
  Constant32 : Constant  Value=137  OutDataTypeStr=double
  Demux1 : Demux  Outputs=28
  Demux2 : Demux  Outputs=16
  FrameByteEnd : Constant  Value=126  OutDataTypeStr=uint8
  FrameByteStart : Constant  Value=126  OutDataTypeStr=uint8
  Framing byte : Constant  Value=68  OutDataTypeStr=uint8
  General CRC Generator1 : commcrc2/General CRC Generator  genPoly=[1 0 0 0 1 0 0 0 0 0 0 1 0 0 0 0 1]  iniStates=0  directMethod=off  reflectInputBytes=off  reflectChecksums=off  finalXOR=0  numChecksums=1
  Integer to Bit Converter{,1..25} (26 alike) : commutil2/Integer to Bit Converter  nbits=8  signedInputValues=Unsigned  bitOrder=MSB first  outDtype=boolean
  Mux1 : Mux  Inputs=26
  Mux2 : Mux  Inputs=30
  SerialFrame : Outport
  wires:
  Bit to Integer Converter27/1 -> Mux2/3
  Demux1/28 -> Bit to Integer Converter27/1
  FrameByteStart/1 -> Mux2/30
  Bit to Integer Converter26/1 -> Mux2/2
  Demux1/27 -> Bit to Integer Converter26/1
  Demux1/15 -> Bit to Integer Converter18/1
  Demux1/14 -> Bit to Integer Converter13/1
  Demux1/6 -> Bit to Integer Converter5/1
  Demux1/16 -> Bit to Integer Converter19/1
  Demux1/25 -> Bit to Integer Converter22/1
  Demux1/17 -> Bit to Integer Converter14/1
  Demux1/18 -> Bit to Integer Converter15/1
  Demux1/26 -> Bit to Integer Converter23/1
  Demux1/22 -> Bit to Integer Converter25/1
  Demux1/23 -> Bit to Integer Converter20/1
  Demux1/20 -> Bit to Integer Converter17/1
  Demux1/19 -> Bit to Integer Converter16/1
  Demux1/5 -> Bit to Integer Converter4/1
  Demux1/21 -> Bit to Integer Converter24/1
  Demux1/4 -> Bit to Integer Converter3/1
  Demux1/24 -> Bit to Integer Converter21/1
  Constant31/1 -> Integer to Bit Converter7/1
  Integer to Bit Converter19/1 -> Mux1/20
  Integer to Bit Converter20/1 -> Mux1/21
  Integer to Bit Converter9/1 -> Mux1/10
  Integer to Bit Converter18/1 -> Mux1/19
  Demux1/12 -> Bit to Integer Converter11/1
  Mux2/1 -> SerialFrame/1
  Integer to Bit Converter12/1 -> Mux1/13
  Demux2/9 -> Integer to Bit Converter18/1
  Demux1/7 -> Bit to Integer Converter6/1
  Demux1/13 -> Bit to Integer Converter12/1
  Demux1/9 -> Bit to Integer Converter8/1
  Demux1/1 -> Bit to Integer Converter/1
  Demux2/11 -> Integer to Bit Converter20/1
  Demux1/11 -> Bit to Integer Converter10/1
  AM Packet type/1 -> Integer to Bit Converter9/1
  FrameByteEnd/1 -> Mux2/1
  Integer to Bit Converter22/1 -> Mux1/23
  Integer to Bit Converter21/1 -> Mux1/22
  Integer to Bit Converter25/1 -> Mux1/26
  Constant32/1 -> Integer to Bit Converter8/1
  Integer to Bit Converter8/1 -> Mux1/9
  General CRC Generator1/1 -> Demux1/1
  Integer to Bit Converter7/1 -> Mux1/8
  Demux1/3 -> Bit to Integer Converter2/1
  Integer to Bit Converter2/1 -> Mux1/3
  Integer to Bit Converter3/1 -> Mux1/4
  Constant28/1 -> Integer to Bit Converter4/1
  Integer to Bit Converter4/1 -> Mux1/5
  Constant27/1 -> Integer to Bit Converter3/1
  Constant26/1 -> Integer to Bit Converter2/1
  Constant29/1 -> Integer to Bit Converter5/1
  Integer to Bit Converter1/1 -> Mux1/2
  Integer to Bit Converter5/1 -> Mux1/6
  Demux2/14 -> Integer to Bit Converter23/1
  Demux2/16 -> Integer to Bit Converter25/1
  Mux1/1 -> General CRC Generator1/1
  Framing byte/1 -> Integer to Bit Converter/1
  Demux2/15 -> Integer to Bit Converter24/1
  Demux2/13 -> Integer to Bit Converter22/1
  Integer to Bit Converter/1 -> Mux1/1
  Demux2/12 -> Integer to Bit Converter21/1
  Constant25/1 -> Integer to Bit Converter1/1
  Demux2/8 -> Integer to Bit Converter17/1
  Integer to Bit Converter10/1 -> Mux1/11
  Demux2/10 -> Integer to Bit Converter19/1
  Integer to Bit Converter6/1 -> Mux1/7
  Demux1/2 -> Bit to Integer Converter1/1
  Integer to Bit Converter16/1 -> Mux1/17
  Integer to Bit Converter15/1 -> Mux1/16
  Integer to Bit Converter17/1 -> Mux1/18
  Integer to Bit Converter13/1 -> Mux1/14
  Demux1/8 -> Bit to Integer Converter7/1
  Demux1/10 -> Bit to Integer Converter9/1
  Constant30/1 -> Integer to Bit Converter6/1
  Integer to Bit Converter11/1 -> Mux1/12
  Integer to Bit Converter23/1 -> Mux1/24
  Integer to Bit Converter24/1 -> Mux1/25
  Integer to Bit Converter14/1 -> Mux1/15
  Demux2/6 -> Integer to Bit Converter15/1
  Demux2/5 -> Integer to Bit Converter14/1
  Bit to Integer Converter22/1 -> Mux2/5
  SerialData/1 -> Demux2/1
  Bit to Integer Converter21/1 -> Mux2/6
  Demux2/2 -> Integer to Bit Converter11/1
  Demux2/1 -> Integer to Bit Converter10/1
  Bit to Integer Converter17/1 -> Mux2/10
  Bit to Integer Converter20/1 -> Mux2/7
  Bit to Integer Converter/1 -> Mux2/29
  Bit to Integer Converter9/1 -> Mux2/20
  Bit to Integer Converter7/1 -> Mux2/22
  Bit to Integer Converter11/1 -> Mux2/18
  Bit to Integer Converter4/1 -> Mux2/25
  Bit to Integer Converter1/1 -> Mux2/28
  Bit to Integer Converter6/1 -> Mux2/23
  Bit to Integer Converter10/1 -> Mux2/19
  Bit to Integer Converter25/1 -> Mux2/8
  Bit to Integer Converter15/1 -> Mux2/12
  Bit to Integer Converter13/1 -> Mux2/16
  Bit to Integer Converter16/1 -> Mux2/11
  Bit to Integer Converter2/1 -> Mux2/27
  Bit to Integer Converter5/1 -> Mux2/24
  Demux2/7 -> Integer to Bit Converter16/1
  Bit to Integer Converter14/1 -> Mux2/13
  Bit to Integer Converter19/1 -> Mux2/14
  Bit to Integer Converter12/1 -> Mux2/17
  Bit to Integer Converter18/1 -> Mux2/15
  Demux2/3 -> Integer to Bit Converter12/1
  Bit to Integer Converter8/1 -> Mux2/21
  Bit to Integer Converter24/1 -> Mux2/9
  Demux2/4 -> Integer to Bit Converter13/1
  Bit to Integer Converter3/1 -> Mux2/26
  Bit to Integer Converter23/1 -> Mux2/4

== system Control_Loop4_2Model/GISOO-Simulation Environment/SkyMote3/Triggered Subsystem ==
  In2 : Inport
  Trigger : TriggerPort
  Byte Reversal1 : etargetslib/Byte Reversal  numInp=1
  Data Type Conversion1 : DataTypeConversion  OutDataTypeStr=uint32
  Pack : xpclib/UDP/Pack  datatypes={'uint32'}  byteAlign=1
  UDP Send : dspnetwork/UDP Send  remoteURL='127.0.0.1'  remotePort=18000+moteID  localURL='0.0.0.0'  localPortSource=Automatically determine  localPort=-1  sampletime=-1  separateLengthPort=0
  wires:
  Data Type Conversion1/1 -> Byte Reversal1/1
  Byte Reversal1/1 -> Pack/1
  Pack/1 -> UDP Send/1
  In2/1 -> Data Type Conversion1/1

== system Control_Loop4_2Model/GISOO-Simulation Environment/SkyMote3/Triggered Subsystem1 ==
  In2 : Inport
  Trigger : TriggerPort
  Byte Reversal1 : etargetslib/Byte Reversal  numInp=1
  Data Type Conversion1 : DataTypeConversion  OutDataTypeStr=uint32
  Pack : xpclib/UDP/Pack  datatypes={'uint32'}  byteAlign=1
  UDP Send : dspnetwork/UDP Send  remoteURL='127.0.0.1'  remotePort=18000+moteID  localURL='0.0.0.0'  localPortSource=Automatically determine  localPort=-1  sampletime=-1  separateLengthPort=0
  wires:
  Byte Reversal1/1 -> Pack/1
  Data Type Conversion1/1 -> Byte Reversal1/1
  In2/1 -> Data Type Conversion1/1
  Pack/1 -> UDP Send/1

== system Control_Loop4_2Model/GISOO-Simulation Environment/SkyMote3/Triggered Subsystem2 ==
  In2 : Inport
  Trigger : TriggerPort
  Byte Reversal : etargetslib/Byte Reversal  numInp=1
  Data Type Conversion1 : DataTypeConversion  OutDataTypeStr=uint32
  Pack : xpclib/UDP/Pack  datatypes={'uint32'}  byteAlign=1
  UDP Send : dspnetwork/UDP Send  remoteURL='127.0.0.1'  remotePort=18000+moteID  localURL='0.0.0.0'  localPortSource=Automatically determine  localPort=-1  sampletime=-1  separateLengthPort=0
  Out1 : Outport
  wires:
  Byte Reversal/1 -> Pack/1
  Pack/1 -> UDP Send/1
  Data Type Conversion1/1 -> Byte Reversal/1, Out1/1
  In2/1 -> Data Type Conversion1/1

== system Control_Loop4_2Model/GISOO-Simulation Environment/SkyMote3/Triggered Subsystem3 ==
  In2 : Inport
  Trigger : TriggerPort
  Byte Reversal : etargetslib/Byte Reversal  numInp=1
  Data Type Conversion1 : DataTypeConversion  OutDataTypeStr=uint32
  Pack : xpclib/UDP/Pack  datatypes={'uint32'}  byteAlign=1
  UDP Send : dspnetwork/UDP Send  remoteURL='127.0.0.1'  remotePort=18000+moteID  localURL='0.0.0.0'  localPortSource=Automatically determine  localPort=-1  sampletime=-1  separateLengthPort=0
  Out1 : Outport
  wires:
  Byte Reversal/1 -> Pack/1
  In2/1 -> Data Type Conversion1/1
  Data Type Conversion1/1 -> Out1/1, Byte Reversal/1
  Pack/1 -> UDP Send/1
